simulink model "quadcopter_dynamics"  (R2016b)
settings: Solver=VariableStepAuto  StartTime=0.0  StopTime=10.0  RelTol=1e-3
undefined symbols (not defined in the file): dist_to_cg_y, ft, gravity, Ixx, Iyy, Izz, k_drag, k_thrust, lbs, mass_quad, pitch_inertia_ratio, roll_inertia_ratio, sec, yaw_inertia_ratio
settings Model: Creator=aaronniemiec  LastModifiedBy=aaronniemiec

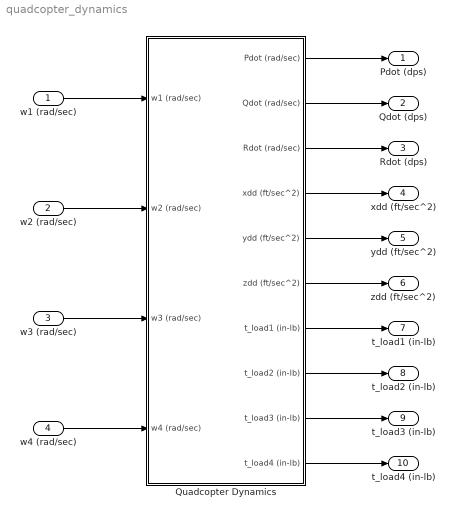
== system quadcopter_dynamics ==
  w1 (rad/sec) : Inport
  w2 (rad/sec) : Inport  Port=2
  w3 (rad/sec) : Inport  Port=3
  "w4 (rad/sec) " : Inport  Port=4
  Quadcopter Dynamics : Subsystem
  Pdot (dps) : Outport
  Qdot (dps) : Outport  Port=2
  Rdot (dps) : Outport  Port=3
  xdd (ft/sec^2) : Outport  Port=4
  ydd (ft/sec^2) : Outport  Port=5
  zdd (ft/sec^2) : Outport  Port=6
  t_load1 (in-lb) : Outport  Port=7
  t_load2 (in-lb) : Outport  Port=8
  t_load3 (in-lb) : Outport  Port=9
  t_load4 (in-lb) : Outport  Port=10
  wires:
  w1 (rad/sec)/1 -> Quadcopter Dynamics/1(w1 (rad/sec))
  w2 (rad/sec)/1 -> Quadcopter Dynamics/2(w2 (rad/sec))
  w3 (rad/sec)/1 -> Quadcopter Dynamics/3(w3 (rad/sec))
  "w4 (rad/sec) "/1 -> Quadcopter Dynamics/4("w4 (rad/sec) ")
  Quadcopter Dynamics/7(t_load1 (in-lb)) -> t_load1 (in-lb)/1
  Quadcopter Dynamics/8(t_load2 (in-lb)) -> t_load2 (in-lb)/1
  Quadcopter Dynamics/9(t_load3 (in-lb)) -> t_load3 (in-lb)/1
  Quadcopter Dynamics/10("t_load4 (in-lb) ") -> t_load4 (in-lb)/1
  Quadcopter Dynamics/1(Pdot (rad/sec)) -> Pdot (dps)/1
  Quadcopter Dynamics/2(Qdot (rad/sec)) -> Qdot (dps)/1
  Quadcopter Dynamics/3(Rdot (rad/sec)) -> Rdot (dps)/1
  Quadcopter Dynamics/4(xdd (ft/sec^2)) -> xdd (ft/sec^2)/1
  Quadcopter Dynamics/5(ydd (ft/sec^2)) -> ydd (ft/sec^2)/1
  Quadcopter Dynamics/6(zdd (ft/sec^2)) -> zdd (ft/sec^2)/1

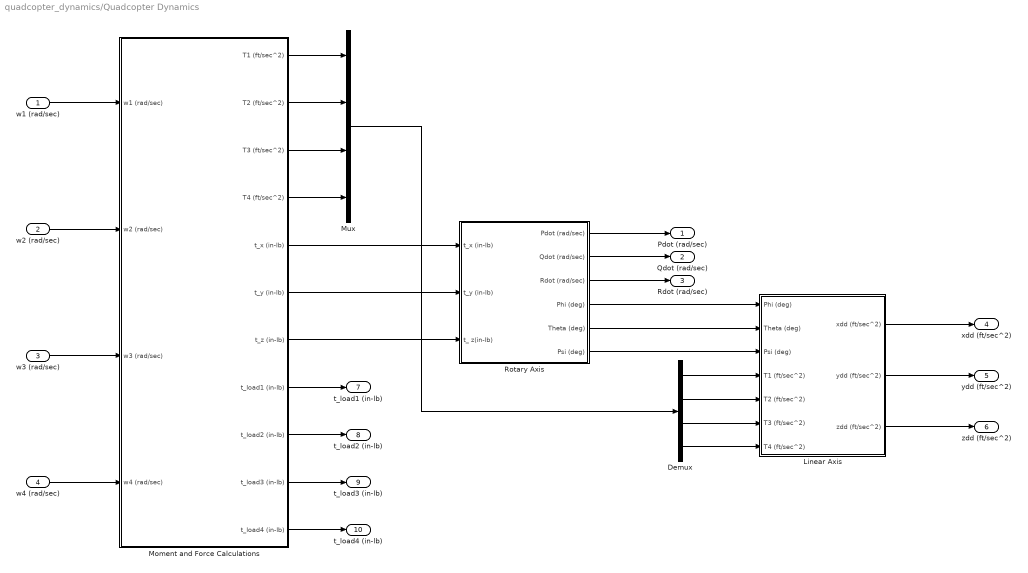
== system quadcopter_dynamics/Quadcopter Dynamics ==
  w1 (rad/sec) : Inport
  w2 (rad/sec) : Inport  Port=2
  w3 (rad/sec) : Inport  Port=3
  "w4 (rad/sec) " : Inport  Port=4
  Demux : Demux
  Linear Axis : Subsystem
  Moment and Force Calculations : Subsystem
  Mux : Mux
  Rotary Axis : Subsystem
  Pdot (rad/sec) : Outport
  Qdot (rad/sec) : Outport  Port=2
  Rdot (rad/sec) : Outport  Port=3
  xdd (ft/sec^2) : Outport  Port=4
  ydd (ft/sec^2) : Outport  Port=5
  zdd (ft/sec^2) : Outport  Port=6
  t_load1 (in-lb) : Outport  Port=7
  t_load2 (in-lb) : Outport  Port=8
  t_load3 (in-lb) : Outport  Port=9
  "t_load4 (in-lb) " : Outport  Port=10
  wires:
  Moment and Force Calculations/5(t_x (in-lb)) -> Rotary Axis/1(t_x (in-lb))
  Moment and Force Calculations/6(t_y (in-lb)) -> Rotary Axis/2(t_y (in-lb))
  Moment and Force Calculations/7(t_z (in-lb)) -> Rotary Axis/3(t_ z(in-lb))
  Rotary Axis/4(Phi (deg)) -> Linear Axis/1(Phi (deg))
  Rotary Axis/5(Theta (deg)) -> Linear Axis/2(Theta (deg))
  Rotary Axis/6(Psi (deg)) -> Linear Axis/3(Psi (deg))
  w1 (rad/sec)/1 -> Moment and Force Calculations/1(w1 (rad/sec))
  w2 (rad/sec)/1 -> Moment and Force Calculations/2(w2 (rad/sec))
  w3 (rad/sec)/1 -> Moment and Force Calculations/3(w3 (rad/sec))
  "w4 (rad/sec) "/1 -> Moment and Force Calculations/4("w4 (rad/sec) ")
  Moment and Force Calculations/8(t_load1 (in-lb)) -> t_load1 (in-lb)/1
  Moment and Force Calculations/9(t_load2 (in-lb)) -> t_load2 (in-lb)/1
  Moment and Force Calculations/10(t_load3 (in-lb)) -> t_load3 (in-lb)/1
  Moment and Force Calculations/11("t_load4 (in-lb) ") -> "t_load4 (in-lb) "/1
  Rotary Axis/3(Rdot (rad/sec)) -> Rdot (rad/sec)/1
  Rotary Axis/2(Qdot (rad/sec)) -> Qdot (rad/sec)/1
  Rotary Axis/1(Pdot (rad/sec)) -> Pdot (rad/sec)/1
  Linear Axis/1(xdd (ft/sec^2)) -> xdd (ft/sec^2)/1
  Linear Axis/2(ydd (ft/sec^2)) -> ydd (ft/sec^2)/1
  Linear Axis/3(zdd (ft/sec^2)) -> zdd (ft/sec^2)/1
  Moment and Force Calculations/1(T1 (ft/sec^2)) -> Mux/1
  Moment and Force Calculations/2(T2 (ft/sec^2)) -> Mux/2
  Moment and Force Calculations/3(T3 (ft/sec^2)) -> Mux/3
  Moment and Force Calculations/4(T4 (ft/sec^2)) -> Mux/4
  Mux/1 -> Demux/1
  Demux/3 -> Linear Axis/6(T3 (ft/sec^2))
  Demux/4 -> Linear Axis/7(T4 (ft/sec^2))
  Demux/2 -> Linear Axis/5(T2 (ft/sec^2))
  Demux/1 -> Linear Axis/4(T1 (ft/sec^2))

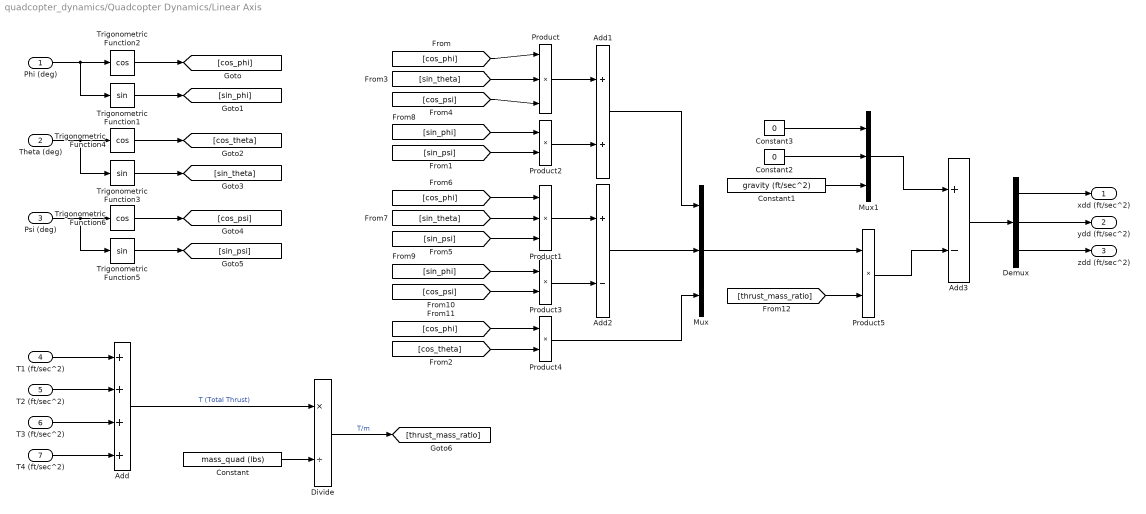
== system quadcopter_dynamics/Quadcopter Dynamics/Linear Axis ==
  Phi (deg) : Inport
  Theta (deg) : Inport  Port=2
  Psi (deg) : Inport  Port=3
  T1 (ft/sec^2) : Inport  Port=4
  T2 (ft/sec^2) : Inport  Port=5
  T3 (ft/sec^2) : Inport  Port=6
  T4 (ft/sec^2) : Inport  Port=7
  Add : Sum  Inputs=4
  Add1 : Sum  Inputs=2
  Add2 : Sum  Inputs=+-
  Add3 : Sum  Inputs=+-
  Constant : Constant  Value=mass_quad (lbs)
  Constant1 : Constant  Value=gravity (ft/sec^2)
  Constant2 : Constant  Value=0
  Constant3 : Constant  Value=0
  Demux : Demux  Outputs=3
  Divide : Product  Inputs=*/
  Mux : Mux  Inputs=3
  Mux1 : Mux  Inputs=3
  Product : Product  Inputs=3
  Product1 : Product  Inputs=3
  Product{2..5} (4 alike) : Product
  Trigonometric Function1 : Trigonometry
  Trigonometric Function2 : Trigonometry  Operator=cos
  Trigonometric Function3 : Trigonometry
  Trigonometric Function4 : Trigonometry  Operator=cos
  Trigonometric Function5 : Trigonometry
  Trigonometric Function6 : Trigonometry  Operator=cos
  xdd (ft/sec^2) : Outport
  ydd (ft/sec^2) : Outport  Port=2
  zdd (ft/sec^2) : Outport  Port=3
  wires:
  T2 (ft/sec^2)/1 -> Add/2
  T3 (ft/sec^2)/1 -> Add/3
  T1 (ft/sec^2)/1 -> Add/1
  T4 (ft/sec^2)/1 -> Add/4
  Phi (deg)/1 -> Trigonometric Function1/1, Trigonometric Function2/1
  Theta (deg)/1 -> Trigonometric Function3/1, Trigonometric Function4/1
  Psi (deg)/1 -> Trigonometric Function5/1, Trigonometric Function6/1
  Add/1 -> Divide/1  "T (Total Thrust)"
  Constant/1 -> Divide/2
  Trigonometric Function2/1 -> [cos_phi]
  Trigonometric Function4/1 -> [cos_theta]
  Trigonometric Function3/1 -> [sin_theta]
  Trigonometric Function6/1 -> [cos_psi]
  Trigonometric Function5/1 -> [sin_psi]
  Trigonometric Function1/1 -> [sin_phi]
  [cos_phi] -> Product/1
  [cos_psi] -> Product/3
  Product/1 -> Add1/1
  [sin_phi] -> Product2/1
  [sin_psi] -> Product2/2
  Product2/1 -> Add1/2
  [sin_theta] -> Product/2
  [cos_phi] -> Product1/1
  [sin_psi] -> Product1/3
  Product1/1 -> Add2/1
  [sin_phi] -> Product3/1
  Product3/1 -> Add2/2
  [sin_theta] -> Product1/2
  [cos_psi] -> Product3/2
  Divide/1 -> [thrust_mass_ratio]  "T/m"
  [cos_theta] -> Product4/2
  [cos_phi] -> Product4/1
  Product4/1 -> Mux/3
  Add1/1 -> Mux/1
  Add2/1 -> Mux/2
  [thrust_mass_ratio] -> Product5/2
  Mux/1 -> Product5/1
  Constant3/1 -> Mux1/1
  Constant2/1 -> Mux1/2
  Constant1/1 -> Mux1/3
  Demux/1 -> xdd (ft/sec^2)/1
  Demux/3 -> zdd (ft/sec^2)/1
  Demux/2 -> ydd (ft/sec^2)/1
  Add3/1 -> Demux/1
  Product5/1 -> Add3/2
  Mux1/1 -> Add3/1

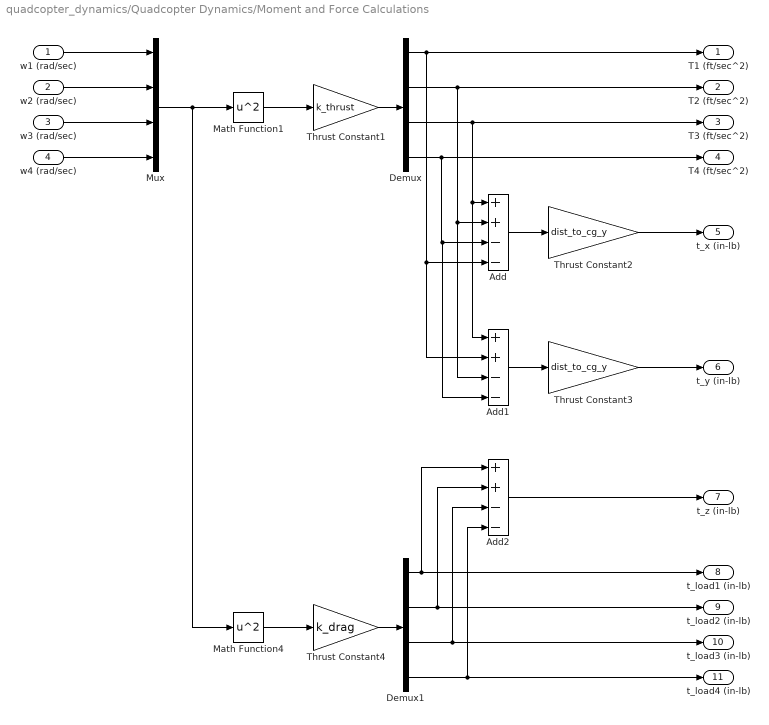
== system quadcopter_dynamics/Quadcopter Dynamics/Moment and Force Calculations ==
  w1 (rad/sec) : Inport
  w2 (rad/sec) : Inport  Port=2
  w3 (rad/sec) : Inport  Port=3
  "w4 (rad/sec) " : Inport  Port=4
  Add : Sum  Inputs=++--
  Add1 : Sum  Inputs=++--
  Add2 : Sum  Inputs=++--
  Demux : Demux
  Demux1 : Demux
  Math Function1 : Math  Operator=square  SaturateOnIntegerOverflow=on
  Math Function4 : Math  Operator=square  SaturateOnIntegerOverflow=on
  Mux : Mux
  Thrust Constant1 : Gain  Gain=k_thrust
  Thrust Constant2 : Gain  Gain=dist_to_cg_y
  Thrust Constant3 : Gain  Gain=dist_to_cg_y
  Thrust Constant4 : Gain  Gain=k_drag
  T1 (ft/sec^2) : Outport
  T2 (ft/sec^2) : Outport  Port=2
  T3 (ft/sec^2) : Outport  Port=3
  T4 (ft/sec^2) : Outport  Port=4
  t_x (in-lb) : Outport  Port=5
  t_y (in-lb) : Outport  Port=6
  t_z (in-lb) : Outport  Port=7
  t_load1 (in-lb) : Outport  Port=8
  t_load2 (in-lb) : Outport  Port=9
  t_load3 (in-lb) : Outport  Port=10
  "t_load4 (in-lb) " : Outport  Port=11
  wires:
  Math Function1/1 -> Thrust Constant1/1
  Math Function4/1 -> Thrust Constant4/1
  Thrust Constant4/1 -> Demux1/1
  Thrust Constant1/1 -> Demux/1
  Mux/1 -> Math Function4/1, Math Function1/1
  Demux/2 -> T2 (ft/sec^2)/1, Add1/3, Add/2
  Demux/4 -> T4 (ft/sec^2)/1, Add1/4, Add/3
  w1 (rad/sec)/1 -> Mux/1
  w2 (rad/sec)/1 -> Mux/2
  w3 (rad/sec)/1 -> Mux/3
  "w4 (rad/sec) "/1 -> Mux/4
  Demux1/2 -> t_load2 (in-lb)/1, Add2/2
  Demux1/1 -> t_load1 (in-lb)/1, Add2/1
  Demux1/4 -> "t_load4 (in-lb) "/1, Add2/4
  Demux1/3 -> t_load3 (in-lb)/1, Add2/3
  Demux/3 -> T3 (ft/sec^2)/1, Add1/1, Add/1
  Add/1 -> Thrust Constant2/1
  Demux/1 -> T1 (ft/sec^2)/1, Add1/2, Add/4
  Add1/1 -> Thrust Constant3/1
  Add2/1 -> t_z (in-lb)/1
  Thrust Constant3/1 -> t_y (in-lb)/1
  Thrust Constant2/1 -> t_x (in-lb)/1

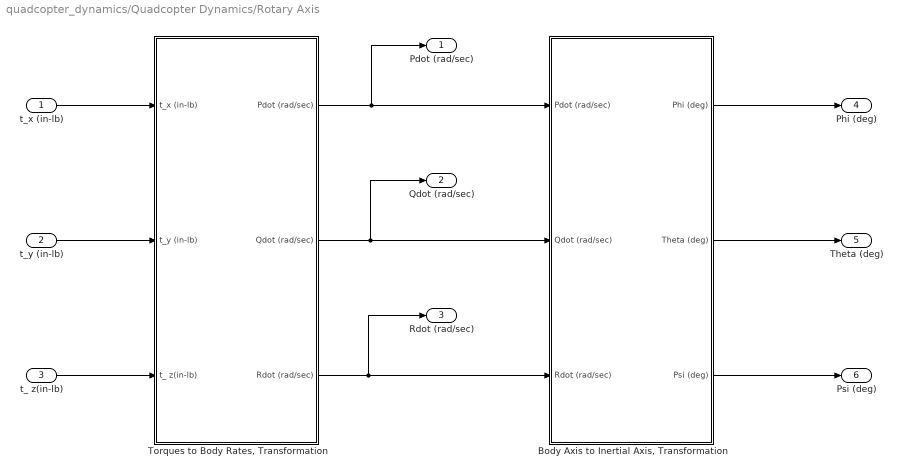
== system quadcopter_dynamics/Quadcopter Dynamics/Rotary Axis ==
  t_x (in-lb) : Inport
  t_y (in-lb) : Inport  Port=2
  t_ z(in-lb) : Inport  Port=3
  "Body Axis to Inertial Axis, Transformation" : Subsystem
  "Torques to Body Rates, Transformation" : Subsystem
  Pdot (rad/sec) : Outport
  Qdot (rad/sec) : Outport  Port=2
  Rdot (rad/sec) : Outport  Port=3
  Phi (deg) : Outport  Port=4
  Theta (deg) : Outport  Port=5
  Psi (deg) : Outport  Port=6
  wires:
  "Body Axis to Inertial Axis, Transformation"/2(Theta (deg)) -> Theta (deg)/1
  "Body Axis to Inertial Axis, Transformation"/3(Psi (deg)) -> Psi (deg)/1
  "Body Axis to Inertial Axis, Transformation"/1(Phi (deg)) -> Phi (deg)/1
  "Torques to Body Rates, Transformation"/1(Pdot (rad/sec)) -> Pdot (rad/sec)/1, "Body Axis to Inertial Axis, Transformation"/1(Pdot (rad/sec))
  "Torques to Body Rates, Transformation"/2(Qdot (rad/sec)) -> Qdot (rad/sec)/1, "Body Axis to Inertial Axis, Transformation"/2(Qdot (rad/sec))
  "Torques to Body Rates, Transformation"/3(Rdot (rad/sec)) -> Rdot (rad/sec)/1, "Body Axis to Inertial Axis, Transformation"/3(Rdot (rad/sec))
  t_x (in-lb)/1 -> "Torques to Body Rates, Transformation"/1(t_x (in-lb))
  t_y (in-lb)/1 -> "Torques to Body Rates, Transformation"/2(t_y (in-lb))
  t_ z(in-lb)/1 -> "Torques to Body Rates, Transformation"/3(t_ z(in-lb))

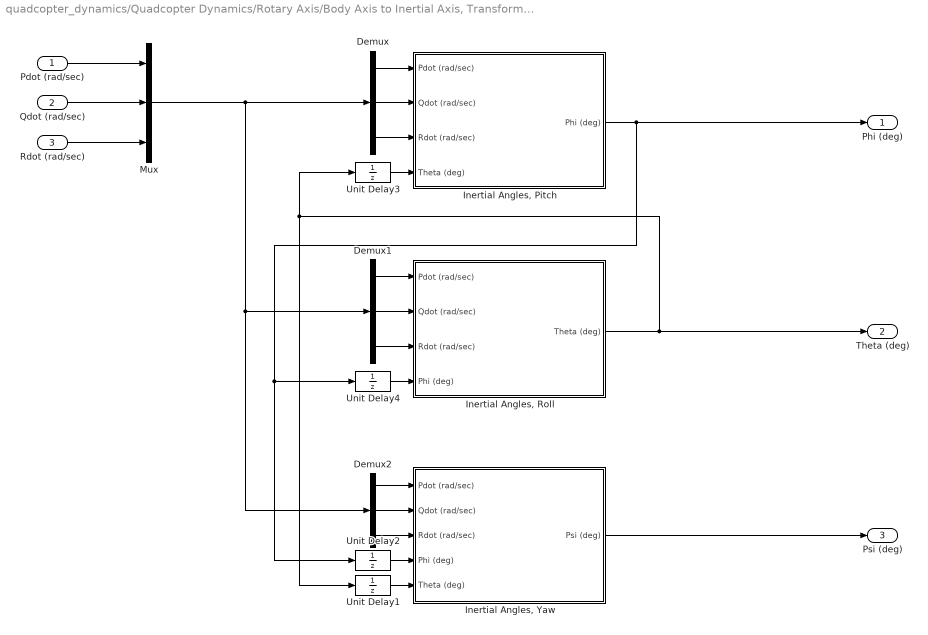
== system quadcopter_dynamics/Quadcopter Dynamics/Rotary Axis/Body Axis to Inertial Axis, Transformation ==
  Pdot (rad/sec) : Inport
  Qdot (rad/sec) : Inport  Port=2
  Rdot (rad/sec) : Inport  Port=3
  Demux : Demux  Outputs=3
  Demux1 : Demux  Outputs=3
  Demux2 : Demux  Outputs=3
  "Inertial Angles, Pitch" : Subsystem
  "Inertial Angles, Roll" : Subsystem
  "Inertial Angles, Yaw" : Subsystem
  Mux : Mux  Inputs=3
  Unit Delay{1..4} (4 alike) : UnitDelay  SampleTime=-1
  Phi (deg) : Outport
  Theta (deg) : Outport  Port=2
  Psi (deg) : Outport  Port=3
  wires:
  Rdot (rad/sec)/1 -> Mux/3
  Qdot (rad/sec)/1 -> Mux/2
  Pdot (rad/sec)/1 -> Mux/1
  Mux/1 -> Demux/1, Demux2/1, Demux1/1
  Demux/2 -> "Inertial Angles, Pitch"/2(Qdot (rad/sec))
  Demux/1 -> "Inertial Angles, Pitch"/1(Pdot (rad/sec))
  Demux/3 -> "Inertial Angles, Pitch"/3(Rdot (rad/sec))
  Demux1/2 -> "Inertial Angles, Roll"/2(Qdot (rad/sec))
  Demux1/3 -> "Inertial Angles, Roll"/3(Rdot (rad/sec))
  Demux1/1 -> "Inertial Angles, Roll"/1(Pdot (rad/sec))
  Demux2/2 -> "Inertial Angles, Yaw"/2(Qdot (rad/sec))
  Demux2/3 -> "Inertial Angles, Yaw"/3(Rdot (rad/sec))
  Demux2/1 -> "Inertial Angles, Yaw"/1(Pdot (rad/sec))
  "Inertial Angles, Pitch"/1(Phi (deg)) -> Phi (deg)/1, Unit Delay4/1, Unit Delay2/1
  "Inertial Angles, Roll"/1(Theta (deg)) -> Theta (deg)/1, Unit Delay3/1, Unit Delay1/1
  "Inertial Angles, Yaw"/1(Psi (deg)) -> Psi (deg)/1
  Unit Delay4/1 -> "Inertial Angles, Roll"/4(Phi (deg))
  Unit Delay1/1 -> "Inertial Angles, Yaw"/5(Theta (deg))
  Unit Delay2/1 -> "Inertial Angles, Yaw"/4(Phi (deg))
  Unit Delay3/1 -> "Inertial Angles, Pitch"/4(Theta (deg))

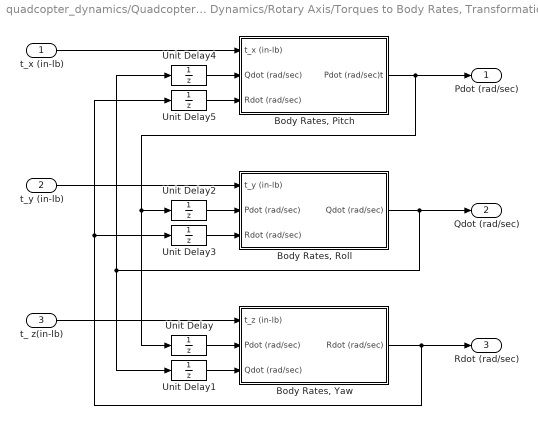
== system quadcopter_dynamics/Quadcopter Dynamics/Rotary Axis/Torques to Body Rates, Transformation ==
  t_x (in-lb) : Inport
  t_y (in-lb) : Inport  Port=2
  t_ z(in-lb) : Inport  Port=3
  "Body Rates, Pitch" : Subsystem
  "Body Rates, Roll" : Subsystem
  "Body Rates, Yaw" : Subsystem
  Unit Delay{,1..5} (6 alike) : UnitDelay  SampleTime=-1
  Pdot (rad/sec) : Outport
  Qdot (rad/sec) : Outport  Port=2
  Rdot (rad/sec) : Outport  Port=3
  wires:
  t_x (in-lb)/1 -> "Body Rates, Pitch"/1(t_x (in-lb))
  t_y (in-lb)/1 -> "Body Rates, Roll"/1(t_y (in-lb))
  t_ z(in-lb)/1 -> "Body Rates, Yaw"/1(t_z (in-lb))
  "Body Rates, Pitch"/1(Pdot (rad/sec)t) -> Pdot (rad/sec)/1, Unit Delay/1, Unit Delay2/1
  "Body Rates, Yaw"/1(Rdot (rad/sec)) -> Rdot (rad/sec)/1, Unit Delay3/1, Unit Delay5/1
  "Body Rates, Roll"/1(Qdot (rad/sec)) -> Qdot (rad/sec)/1, Unit Delay1/1, Unit Delay4/1
  Unit Delay4/1 -> "Body Rates, Pitch"/2(Qdot (rad/sec))
  Unit Delay5/1 -> "Body Rates, Pitch"/3(Rdot (rad/sec))
  Unit Delay2/1 -> "Body Rates, Roll"/2(Pdot (rad/sec))
  Unit Delay3/1 -> "Body Rates, Roll"/3(Rdot (rad/sec))
  Unit Delay/1 -> "Body Rates, Yaw"/2(Pdot (rad/sec))
  Unit Delay1/1 -> "Body Rates, Yaw"/3(Qdot (rad/sec))

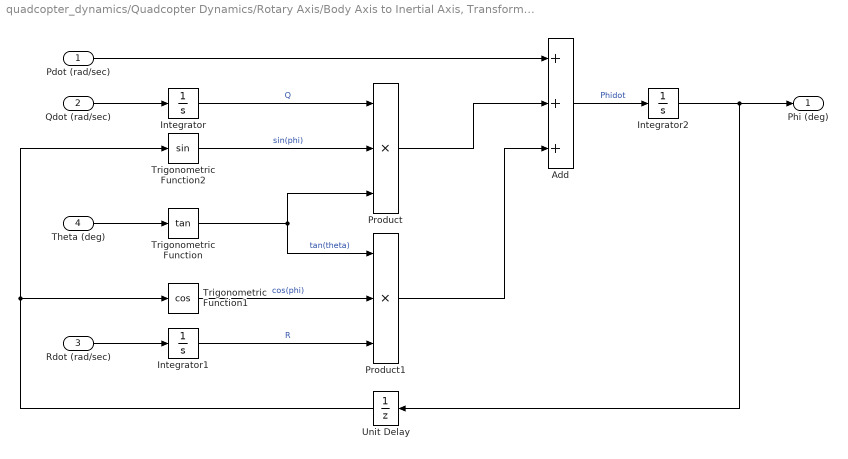
== system quadcopter_dynamics/Quadcopter Dynamics/Rotary Axis/Body Axis to Inertial Axis, Transformation/Inertial Angles, Pitch ==
  Pdot (rad/sec) : Inport
  Qdot (rad/sec) : Inport  Port=2
  Rdot (rad/sec) : Inport  Port=3
  Theta (deg) : Inport  Port=4
  Add : Sum  Inputs=3
  Integrator : Integrator
  Integrator1 : Integrator
  Integrator2 : Integrator
  Product : Product  Inputs=3
  Product1 : Product  Inputs=3
  Trigonometric Function : Trigonometry  Operator=tan
  Trigonometric Function1 : Trigonometry  Operator=cos
  Trigonometric Function2 : Trigonometry
  Unit Delay : UnitDelay  SampleTime=-1
  Phi (deg) : Outport
  wires:
  Pdot (rad/sec)/1 -> Add/1
  Theta (deg)/1 -> Trigonometric Function/1
  Trigonometric Function/1 -> Product/3, Product1/1  "tan(theta)"
  Add/1 -> Integrator2/1  "Phidot"
  Qdot (rad/sec)/1 -> Integrator/1
  Integrator/1 -> Product/1  "Q"
  Rdot (rad/sec)/1 -> Integrator1/1
  Integrator1/1 -> Product1/3  "R"
  Trigonometric Function2/1 -> Product/2  "sin(phi)"
  Trigonometric Function1/1 -> Product1/2  "cos(phi)"
  Product/1 -> Add/2
  Product1/1 -> Add/3
  Unit Delay/1 -> Trigonometric Function2/1, Trigonometric Function1/1
  Integrator2/1 -> Unit Delay/1, Phi (deg)/1

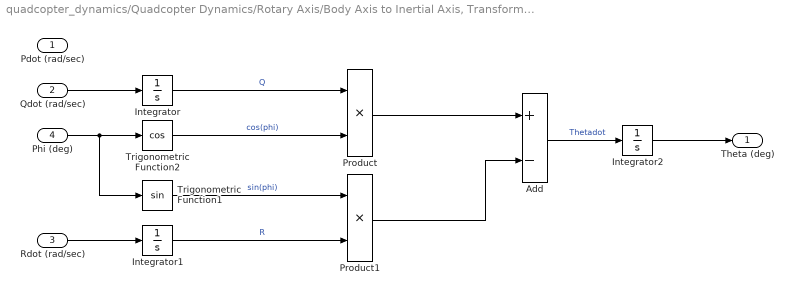
== system quadcopter_dynamics/Quadcopter Dynamics/Rotary Axis/Body Axis to Inertial Axis, Transformation/Inertial Angles, Roll ==
  Pdot (rad/sec) : Inport
  Qdot (rad/sec) : Inport  Port=2
  Rdot (rad/sec) : Inport  Port=3
  Phi (deg) : Inport  Port=4
  Add : Sum  Inputs=+-
  Integrator : Integrator
  Integrator1 : Integrator
  Integrator2 : Integrator
  Product : Product
  Product1 : Product
  Trigonometric Function1 : Trigonometry
  Trigonometric Function2 : Trigonometry  Operator=cos
  Theta (deg) : Outport
  wires:
  Add/1 -> Integrator2/1  "Thetadot"
  Qdot (rad/sec)/1 -> Integrator/1
  Integrator/1 -> Product/1  "Q"
  Rdot (rad/sec)/1 -> Integrator1/1
  Integrator1/1 -> Product1/2  "R"
  Trigonometric Function2/1 -> Product/2  "cos(phi)"
  Trigonometric Function1/1 -> Product1/1  "sin(phi)"
  Product/1 -> Add/1
  Product1/1 -> Add/2
  Phi (deg)/1 -> Trigonometric Function1/1, Trigonometric Function2/1
  Integrator2/1 -> Theta (deg)/1

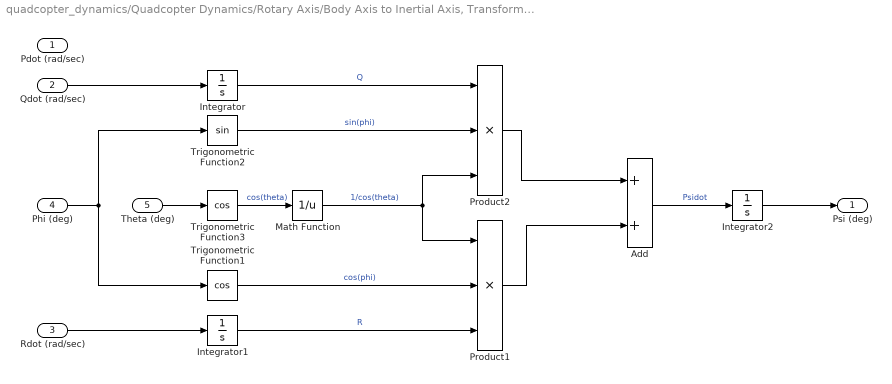
== system quadcopter_dynamics/Quadcopter Dynamics/Rotary Axis/Body Axis to Inertial Axis, Transformation/Inertial Angles, Yaw ==
  Pdot (rad/sec) : Inport
  Qdot (rad/sec) : Inport  Port=2
  Rdot (rad/sec) : Inport  Port=3
  Phi (deg) : Inport  Port=4
  Theta (deg) : Inport  Port=5
  Add : Sum  Inputs=2
  Integrator : Integrator
  Integrator1 : Integrator
  Integrator2 : Integrator
  Math Function : Math  Operator=reciprocal  SaturateOnIntegerOverflow=on
  Product1 : Product  Inputs=3
  Product2 : Product  Inputs=3
  Trigonometric Function1 : Trigonometry  Operator=cos
  Trigonometric Function2 : Trigonometry
  Trigonometric Function3 : Trigonometry  Operator=cos
  Psi (deg) : Outport
  wires:
  Add/1 -> Integrator2/1  "Psidot"
  Qdot (rad/sec)/1 -> Integrator/1
  Integrator/1 -> Product2/1  "Q"
  Rdot (rad/sec)/1 -> Integrator1/1
  Integrator1/1 -> Product1/3  "R"
  Trigonometric Function2/1 -> Product2/2  "sin(phi)"
  Trigonometric Function1/1 -> Product1/2  "cos(phi)"
  Product2/1 -> Add/1
  Product1/1 -> Add/2
  Phi (deg)/1 -> Trigonometric Function2/1, Trigonometric Function1/1
  Theta (deg)/1 -> Trigonometric Function3/1
  Trigonometric Function3/1 -> Math Function/1  "cos(theta)"
  Math Function/1 -> Product1/1, Product2/3  "1/cos(theta)"
  Integrator2/1 -> Psi (deg)/1

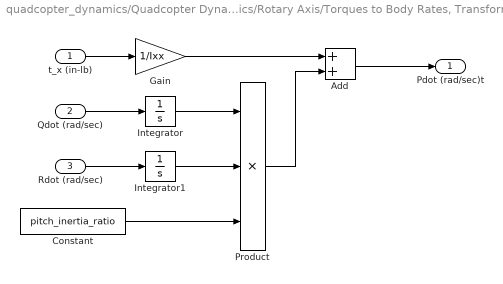
== system quadcopter_dynamics/Quadcopter Dynamics/Rotary Axis/Torques to Body Rates, Transformation/Body Rates, Pitch ==
  t_x (in-lb) : Inport
  Qdot (rad/sec) : Inport  Port=2
  Rdot (rad/sec) : Inport  Port=3
  Add : Sum  Inputs=2
  Constant : Constant  Value=pitch_inertia_ratio
  Gain : Gain  Gain=1/Ixx
  Integrator : Integrator
  Integrator1 : Integrator
  Product : Product  Inputs=3
  Pdot (rad/sec)t : Outport
  wires:
  Qdot (rad/sec)/1 -> Integrator/1
  Rdot (rad/sec)/1 -> Integrator1/1
  Integrator/1 -> Product/1
  Integrator1/1 -> Product/2
  Constant/1 -> Product/3
  Product/1 -> Add/2
  t_x (in-lb)/1 -> Gain/1
  Gain/1 -> Add/1
  Add/1 -> Pdot (rad/sec)t/1

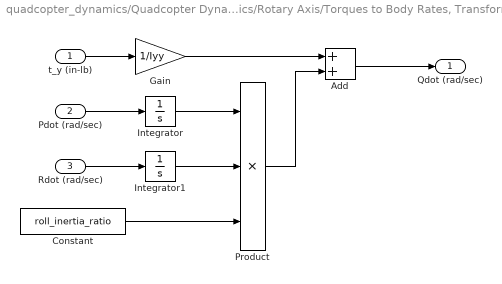
== system quadcopter_dynamics/Quadcopter Dynamics/Rotary Axis/Torques to Body Rates, Transformation/Body Rates, Roll ==
  t_y (in-lb) : Inport
  Pdot (rad/sec) : Inport  Port=2
  Rdot (rad/sec) : Inport  Port=3
  Add : Sum  Inputs=2
  Constant : Constant  Value=roll_inertia_ratio
  Gain : Gain  Gain=1/Iyy
  Integrator : Integrator
  Integrator1 : Integrator
  Product : Product  Inputs=3
  Qdot (rad/sec) : Outport
  wires:
  Pdot (rad/sec)/1 -> Integrator/1
  Rdot (rad/sec)/1 -> Integrator1/1
  Integrator/1 -> Product/1
  Integrator1/1 -> Product/2
  Constant/1 -> Product/3
  Product/1 -> Add/2
  t_y (in-lb)/1 -> Gain/1
  Gain/1 -> Add/1
  Add/1 -> Qdot (rad/sec)/1

== system quadcopter_dynamics/Quadcopter Dynamics/Rotary Axis/Torques to Body Rates, Transformation/Body Rates, Yaw ==
  t_z (in-lb) : Inport
  Pdot (rad/sec) : Inport  Port=2
  Qdot (rad/sec) : Inport  Port=3
  Add : Sum  Inputs=2
  Constant : Constant  Value=yaw_inertia_ratio
  Gain : Gain  Gain=1/Izz
  Integrator : Integrator
  Integrator1 : Integrator
  Product : Product  Inputs=3
  Rdot (rad/sec) : Outport
  wires:
  Pdot (rad/sec)/1 -> Integrator/1
  Qdot (rad/sec)/1 -> Integrator1/1
  Integrator/1 -> Product/1
  Integrator1/1 -> Product/2
  Constant/1 -> Product/3
  Product/1 -> Add/2
  t_z (in-lb)/1 -> Gain/1
  Gain/1 -> Add/1
  Add/1 -> Rdot (rad/sec)/1
